simulink model "development_enviroment2"  (R2022a)
settings: Solver=FixedStepAuto  StartTime=0.0  StopTime=200  FixedStep=0.001  RelTol=1e-3
undefined symbols (not defined in the file): A, B, C, D, k1, k3, k_2, k_2_0, sigbuilder_block, tau_1, tau_1_0, tau_2, tau_2_0, tau_3, tau_3_0, time_to_save_points, zeta, zeta_0
libraries: cstblocks x4
settings Model: Creator=alefr  LastModifiedBy=Alghisi
settings DataIOCC: ReturnWorkspaceOutputs=off
settings DebuggingCC: UnconnectedInputMsg=warning  UnconnectedOutputMsg=warning  UnconnectedLineMsg=warning
settings RTWCC: DLArmComputeVersion=19.05

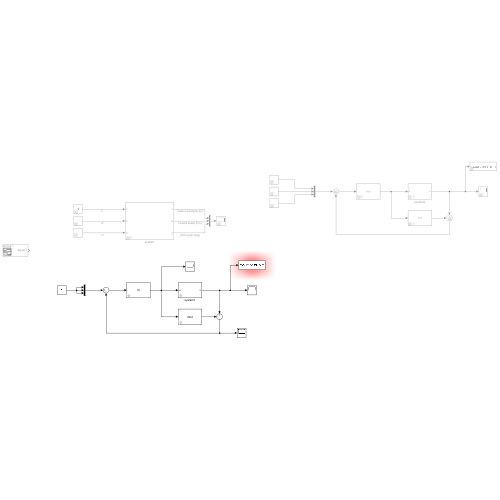
[thumbnail: Simulink's stored preview of the top-level diagram]
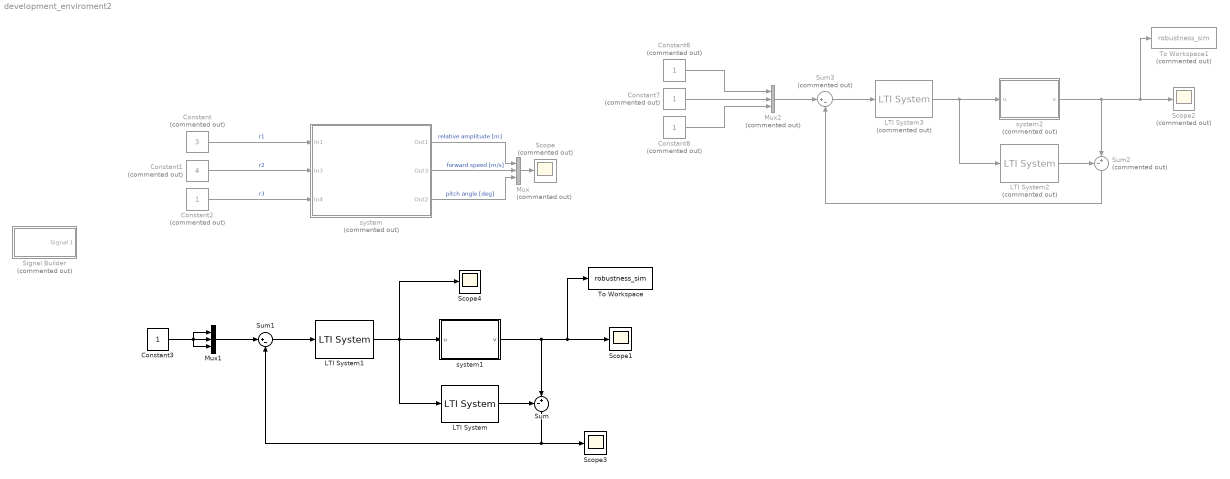
== system development_enviroment2 ==
  Constant : Constant  Commented=on  Value=3
  Constant1 : Constant  Commented=on  Value=4
  Constant{2,6..8} (4 alike) : Constant  Commented=on
  Constant3 : Constant
  LTI System : cstblocks/LTI System  sys=Gtot  IC=[]
  LTI System1 : cstblocks/LTI System  sys=Q  IC=[]
  LTI System2 : cstblocks/LTI System  Commented=on  sys=G  IC=[]
  LTI System3 : cstblocks/LTI System  Commented=on  sys=Q  IC=[]
  Mux : Mux  Commented=on  Inputs=3
  Mux1 : Mux  Inputs=3
  Mux2 : Mux  Commented=on  Inputs=3
  Scope : Scope  Commented=on
  Scope1 : Scope
  Scope2 : Scope  Commented=on
  Scope3 : Scope
  Scope4 : Scope
  Signal Builder : Subsystem  Tag=STV Subsys  Commented=on  LoadFcn=sigbuilder_block('load');  StartFcn=sigbuilder_block('start');  StopFcn=sigbuilder_block('stop');  ClipboardFcn=sigbuilder_block('clipboard');  mask(Sigbuilder block){tuvar=[0:10]}
      mask help: Simulink:masks:SigbuilderBlock_MD
      mask init:
      | if ~strcmp(get_param(bdroot(gcbh),'SimulationStatus'),'stopped') tuvar = sigbuilder_block('maskInit'); end
      settings: CopyFcn=sigbuilder_block('copy');  DeleteFcn=sigbuilder_block('delete');  ModelCloseFcn=sigbuilder_block('modelClose');  PreSaveFcn=sigbuilder_block('preSave');  PauseFcn=sigbuilder_block('pause');  ContinueFcn=sigbuilder_block('continue');  NameChangeFcn=sigbuilder_block('namechange');  OpenFcn=sigbuilder_block('open',[433.8 136.8 550.8 400.2 ]);  CloseFcn=sigbuilder_block('close');
      mask Display: plot(0, 0, 100, 100,[2, 2, 32, 32, 2], [68, 8, 8, 68, 68],[32, 2], [38, 38], [32, 19, 2],[53, 60, 44], [32, 17, 17, 2],[16, 16, 31, 31]);txt = getActiveGroup(gcbh);text(2, 100, txt,'verticalAlignment', 'top');
  Sum : Sum  Inputs=-+|
  Sum1 : Sum  Inputs=|+-
  Sum2 : Sum  Commented=on  Inputs=-+|
  Sum3 : Sum  Commented=on  Inputs=|+-
  To Workspace : ToWorkspace  VariableName=robustness_sim  SaveFormat=Timeseries  SampleTime=time_to_save_points
  To Workspace1 : ToWorkspace  Commented=on  VariableName=robustness_sim  SaveFormat=Timeseries  SampleTime=-1
  system : Subsystem  Commented=on  mask{k_2_param=mean(k_2), tau_1_param=mean(tau_1), tau_2_param=mean(tau_2), zeta_param=mean(zeta), tau_3_param=mean(tau_3)}
      mask prompts: k_2_param "k_2"; tau_1_param "tau_1"; tau_2_param "tau_2"; zeta_param "zeta"; tau_3_param "tau_3"
  system1 : Subsystem  mask{k_2_param=k_2_0, tau_1_param=tau_1_0, tau_2_param=tau_2_0, zeta_param=zeta_0, tau_3_param=tau_3_0}
      mask prompts: k_2_param "k_2"; tau_1_param "tau_1"; tau_2_param "tau_2"; zeta_param "zeta"; tau_3_param "tau_3"
  system2 : Subsystem  Commented=on  mask{k_2_param=mean(k_2), tau_1_param=mean(tau_1), tau_2_param=mean(tau_2), zeta_param=mean(zeta), tau_3_param=mean(tau_3)}
      mask prompts: k_2_param "k_2"; tau_1_param "tau_1"; tau_2_param "tau_2"; zeta_param "zeta"; tau_3_param "tau_3"
  wires:
  Constant/1 -> system/1(In1)  "r1"
  Constant1/1 -> system/2(In3)  "r2"
  Constant2/1 -> system/3(In4)  "r3"
  Mux/1 -> Scope/1
  system/1(Out1) -> Mux/1  "relative amplitude [m]"
  system/3(Out2) -> Mux/3  "pitch angle [deg]"
  system/2(Out3) -> Mux/2  "forward speed [m/s]"
  LTI System1/1 -> LTI System/1, Scope4/1, system1/1(u)
  system1/1(v) -> To Workspace/1, Scope1/1, Sum/2
  LTI System/1 -> Sum/1
  Sum1/1 -> LTI System1/1
  Sum/1 -> Scope3/1, Sum1/2
  Mux1/1 -> Sum1/1
  Constant8/1 -> Mux2/3
  Constant7/1 -> Mux2/2
  Constant6/1 -> Mux2/1
  Mux2/1 -> Sum3/1
  Sum2/1 -> Sum3/2
  Sum3/1 -> LTI System3/1
  LTI System2/1 -> Sum2/1
  system2/1(v) -> To Workspace1/1, Scope2/1, Sum2/2
  LTI System3/1 -> system2/1(u), LTI System2/1
  Constant3/1 -> Mux1/1, Mux1/2, Mux1/3

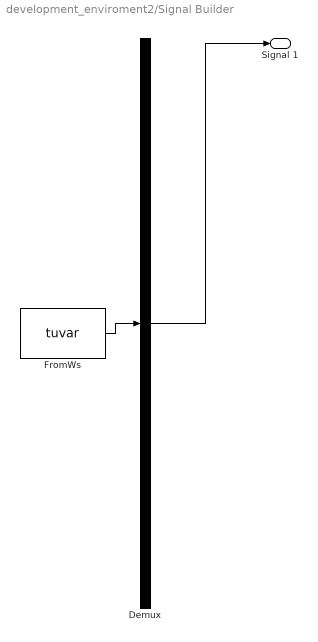
== system development_enviroment2/Signal Builder ==
  Demux : Demux  Tag=STV Demux  Outputs=1
      settings: DisplayOption=none
  FromWs : FromWorkspace  Tag=STV FromWs  VariableName=tuvar
      SigBuilderData=|
      | common.afterFinalStr = 'Extrapolate'
      | common.sampleTime = 0
      | dataSet.timeRange = [0 1000]
      | dataSet.name = 'Group 1'
      | sbobj.Groups.Name = 'Group 1'
      | sbobj.Groups.Signals.Name = 'Signal 1'
      | sbobj.Groups.Signals.XData = [0 20 1000]
      | sbobj.Groups.Signals.YData = [0 1 1]
      | sbobj.Groups.TimeRange = [0 1000]
  Signal 1 : Outport  Tag=STV Outport
  wires:
  Demux/1 -> Signal 1/1
  FromWs/1 -> Demux/1

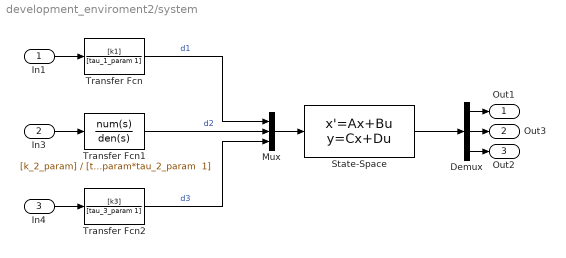
== system development_enviroment2/system ==
  In1 : Inport
  In3 : Inport  Port=2
  In4 : Inport  Port=3
  Demux : Demux  Outputs=3
  Mux : Mux  Inputs=3
  State-Space : StateSpace  A=A  B=B  C=C  D=D  InitialCondition=0  ParameterTunability=Unconstrained
      mask Display: image('plane.png'); % Use "Edit Image" on toolstrip to change.
  Transfer Fcn : TransferFcn  Numerator=[k1]  Denominator=[tau_1_param 1]
  Transfer Fcn1 : TransferFcn  Numerator=[k_2_param]  Denominator="[tau_2_param^2  2*zeta_param*tau_2_param  1]"
  Transfer Fcn2 : TransferFcn  Numerator=[k3]  Denominator=[tau_3_param 1]
  Out1 : Outport
  Out3 : Outport  Port=2
  Out2 : Outport  Port=3
  wires:
  State-Space/1 -> Demux/1
  Transfer Fcn/1 -> Mux/1  "d1"
  Transfer Fcn2/1 -> Mux/3  "d3"
  Transfer Fcn1/1 -> Mux/2  "d2"
  Demux/1 -> Out1/1
  Demux/2 -> Out3/1
  Mux/1 -> State-Space/1
  In4/1 -> Transfer Fcn2/1
  In3/1 -> Transfer Fcn1/1
  In1/1 -> Transfer Fcn/1
  Demux/3 -> Out2/1

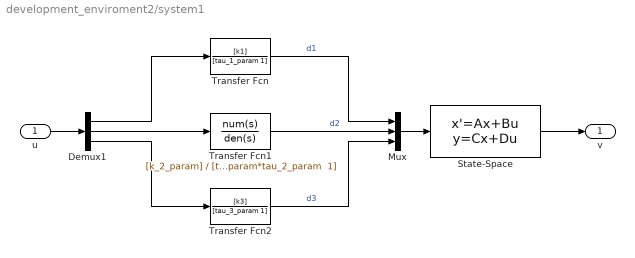
== system development_enviroment2/system1 ==
  u : Inport
  Demux1 : Demux  Outputs=3
  Mux : Mux  Inputs=3
  State-Space : StateSpace  A=A  B=B  C=C  D=D  InitialCondition=0  ParameterTunability=Unconstrained
      mask Display: image('plane.png'); % Use "Edit Image" on toolstrip to change.
  Transfer Fcn : TransferFcn  Numerator=[k1]  Denominator=[tau_1_param 1]
  Transfer Fcn1 : TransferFcn  Numerator=[k_2_param]  Denominator="[tau_2_param^2  2*zeta_param*tau_2_param  1]"
  Transfer Fcn2 : TransferFcn  Numerator=[k3]  Denominator=[tau_3_param 1]
  v : Outport
  wires:
  Demux1/1 -> Transfer Fcn/1
  Demux1/2 -> Transfer Fcn1/1
  Demux1/3 -> Transfer Fcn2/1
  Mux/1 -> State-Space/1
  State-Space/1 -> v/1
  Transfer Fcn1/1 -> Mux/2  "d2"
  Transfer Fcn2/1 -> Mux/3  "d3"
  Transfer Fcn/1 -> Mux/1  "d1"
  u/1 -> Demux1/1

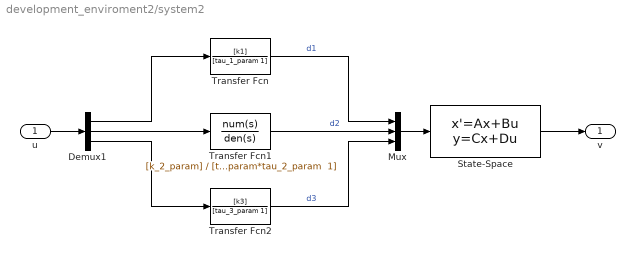
== system development_enviroment2/system2 ==
  u : Inport
  Demux1 : Demux  Outputs=3
  Mux : Mux  Inputs=3
  State-Space : StateSpace  A=A  B=B  C=C  D=D  InitialCondition=0  ParameterTunability=Unconstrained
      mask Display: image('plane.png'); % Use "Edit Image" on toolstrip to change.
  Transfer Fcn : TransferFcn  Numerator=[k1]  Denominator=[tau_1_param 1]
  Transfer Fcn1 : TransferFcn  Numerator=[k_2_param]  Denominator="[tau_2_param^2  2*zeta_param*tau_2_param  1]"
  Transfer Fcn2 : TransferFcn  Numerator=[k3]  Denominator=[tau_3_param 1]
  v : Outport
  wires:
  u/1 -> Demux1/1
  Transfer Fcn/1 -> Mux/1  "d1"
  Transfer Fcn2/1 -> Mux/3  "d3"
  Transfer Fcn1/1 -> Mux/2  "d2"
  State-Space/1 -> v/1
  Mux/1 -> State-Space/1
  Demux1/3 -> Transfer Fcn2/1
  Demux1/2 -> Transfer Fcn1/1
  Demux1/1 -> Transfer Fcn/1
